simulink model "sharedControlWControllers"  (R2018a)
settings: Solver=FixedStepAuto  StartTime=0.0  StopTime=500  FixedStep=.1  RelTol=1e-3
values from neighbouring files (symbols this model uses):
  a = -real(s1) + imag(s1)/tan(angle(s1+b) - theta)    [RLDesignJoystick.m]    (also in gainPlot.m = 10)
  a1 = b1/K    [RLDesignJoystick.m]
  b = 1.2*bb/I    (= 0.4)    [RLDesignJoystick.m]    (also in gainPlot.m)
  b1 = -real(s1)/150    [RLDesignJoystick.m]
  K0 = abs(s1+a)/abs(Gs1)/abs(s1+b)    [RLDesignJoystick.m]    (also in gainPlot.m = 0.5)
  K1 = 1/abs(Gs1)    [RLDesignJoystick.m]
undefined symbols (not defined in the file or in its folder): a2, b2, K2
libraries: simulink x2, commfilt2 x2
settings Model: Creator=transmogrifierlight  LastModifiedBy=thedoctor

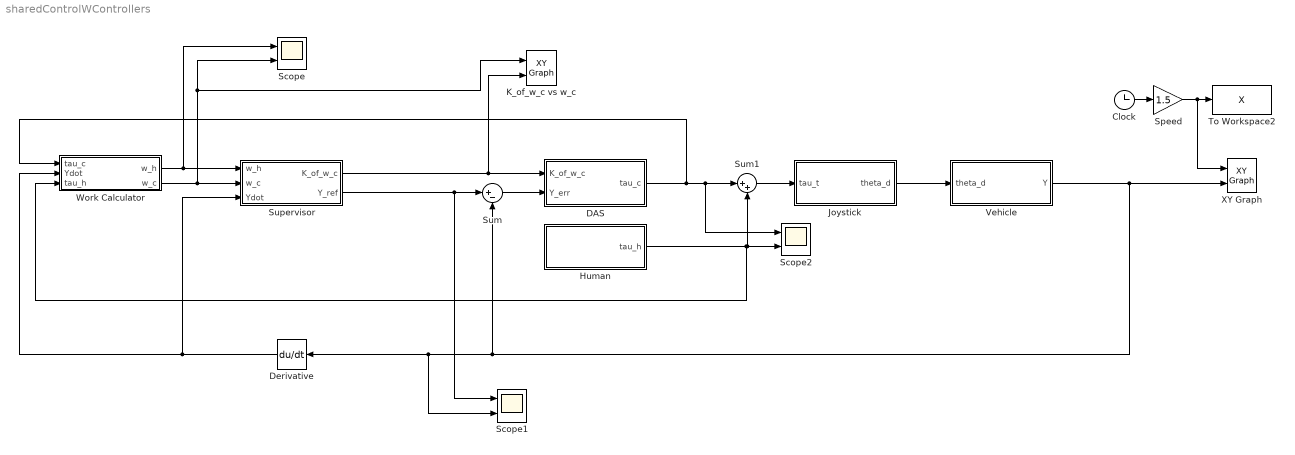
== system sharedControlWControllers ==
  Clock : Clock
  DAS : Subsystem
  Derivative : Derivative
  Human : Subsystem
  Joystick : Subsystem
  K_of_w_c vs w_c : simulink/Sinks/XY Graph  xmin=-01  xmax=2  ymin=-0.5  ymax=1  st=-1
  Scope : Scope  NumInputPorts=2
  Scope1 : Scope  NumInputPorts=2
  Scope2 : Scope  NumInputPorts=2
  Speed : Gain  Gain=1.5
  Sum : Sum  Inputs=|+-
  Sum1 : Sum  Inputs=|++
  Supervisor : Subsystem  mask{gamma_1_sq=0, gamma_2_sq=0, a_d=10, b_d=0.4, sigma_sq=0.3, delta_y=4, K0=0.5}
      mask prompts: gamma_1_sq "DAS Threshold"; gamma_2_sq "Human Threshold"; a_d "a"; b_d "b"; sigma_sq "Lane Change Threshold"; delta_y "Lane Change Delta"
  To Workspace2 : ToWorkspace  VariableName=X  SaveFormat=Timeseries  SampleTime=-1
  Vehicle : Subsystem
  Work Calculator : Subsystem
  XY Graph : simulink/Sinks/XY Graph  xmin=-10  xmax=1.5*1500  ymin=-100  ymax=100  st=-1
  wires:
  Work Calculator/1(w_h) -> Scope/1, Supervisor/1(w_h)
  Work Calculator/2(w_c) -> K_of_w_c vs w_c/1, Scope/2, Supervisor/2(w_c)
  Supervisor/1(K_of_w_c) -> K_of_w_c vs w_c/2, DAS/1("K_of_w_c ")
  Supervisor/2(Y_ref) -> Scope1/1, Sum/1
  Sum/1 -> DAS/2(Y_err)
  DAS/1(tau_c) -> Scope2/1, Sum1/1, Work Calculator/1(tau_c)
  Sum1/1 -> Joystick/1(tau_t)
  Clock/1 -> Speed/1
  Speed/1 -> XY Graph/1, To Workspace2/1
  Vehicle/1(Y) -> Sum/2, Scope1/2, Derivative/1, XY Graph/2
  Derivative/1 -> Supervisor/3(Ydot), Work Calculator/2(Ydot)
  Joystick/1(theta_d) -> Vehicle/1(theta_d)
  Human/1(tau_h) -> Work Calculator/3(tau_h), Sum1/2, Scope2/2

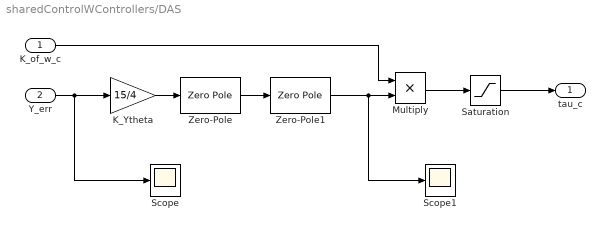
== system sharedControlWControllers/DAS ==
  "K_of_w_c " : Inport
  Y_err : Inport  Port=2
  K_Ytheta : Gain  Gain=15/4
  Multiply : Product
  Saturation : Saturate  UpperLimit=3.5  LowerLimit=-3.5
  Scope : Scope
  Scope1 : Scope
  Zero-Pole : ZeroPole  Zeros=[-b]  Poles=[-a]  Gain=[K0]
  Zero-Pole1 : ZeroPole  Zeros=[-b1]  Poles=[-a1]  Gain=[K1]
  tau_c : Outport
  wires:
  Y_err/1 -> Scope/1, K_Ytheta/1
  Saturation/1 -> tau_c/1
  Multiply/1 -> Saturation/1
  "K_of_w_c "/1 -> Multiply/1
  K_Ytheta/1 -> Zero-Pole/1
  Zero-Pole1/1 -> Scope1/1, Multiply/2
  Zero-Pole/1 -> Zero-Pole1/1

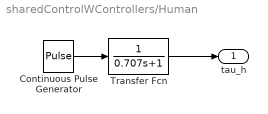
== system sharedControlWControllers/Human ==
  Continuous Pulse Generator : DiscretePulseGenerator  PulseType=Time based  Amplitude=3.5  Period=100  PhaseDelay=30
  Transfer Fcn : TransferFcn  Denominator=[0.707 1]
  tau_h : Outport
  wires:
  Transfer Fcn/1 -> tau_h/1
  Continuous Pulse Generator/1 -> Transfer Fcn/1

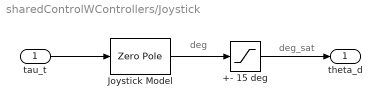
== system sharedControlWControllers/Joystick ==
  note: deg_sat
  note: deg
  tau_t : Inport
  +- 15 deg : Saturate  UpperLimit=15  LowerLimit=-15
  Joystick Model : ZeroPole  Zeros=[]  Poles=[0 -0.254/0.762]  Gain=[0.762]
  theta_d : Outport
  wires:
  Joystick Model/1 -> +- 15 deg/1
  +- 15 deg/1 -> theta_d/1
  tau_t/1 -> Joystick Model/1

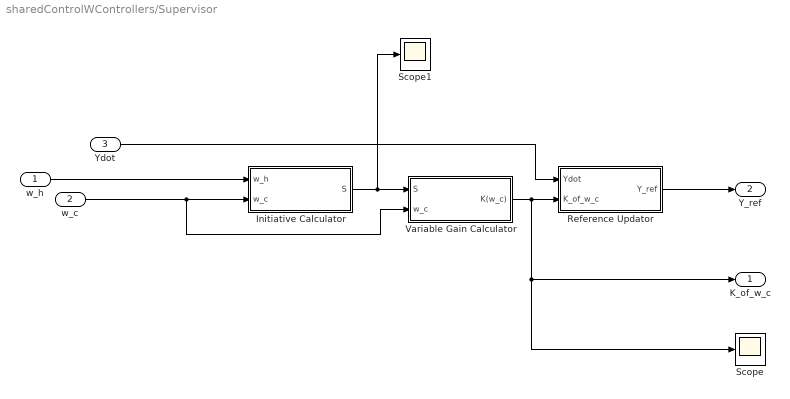
== system sharedControlWControllers/Supervisor ==
  w_h : Inport
  w_c : Inport  Port=2
  Ydot : Inport  Port=3
  Initiative Calculator : Subsystem
  Reference Updator : Subsystem
  Scope : Scope
  Scope1 : Scope
  Variable Gain Calculator : Subsystem
  K_of_w_c : Outport
  Y_ref : Outport  Port=2
  wires:
  w_c/1 -> Variable Gain Calculator/2(w_c), Initiative Calculator/2("w_c ")
  w_h/1 -> Initiative Calculator/1(w_h)
  Initiative Calculator/1(S) -> Scope1/1, Variable Gain Calculator/1(S)
  Variable Gain Calculator/1(K(w_c)) -> Reference Updator/2(K_of_w_c), Scope/1, K_of_w_c/1
  Ydot/1 -> Reference Updator/1(Ydot)
  Reference Updator/1(Y_ref) -> Y_ref/1

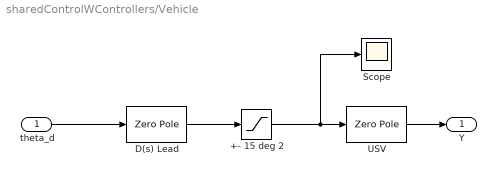
== system sharedControlWControllers/Vehicle ==
  theta_d : Inport
  +- 15 deg 2 : Saturate  UpperLimit=15  LowerLimit=-15
  D(s) Lead : ZeroPole  Zeros=[-b2]  Poles=[-a2]  Gain=[K2]
  Scope : Scope
  USV : ZeroPole  Zeros=[]  Poles=[0 0 -5/4]  Gain=[1.5*1e-2]
  Y : Outport
  wires:
  +- 15 deg 2/1 -> Scope/1, USV/1
  USV/1 -> Y/1
  theta_d/1 -> D(s) Lead/1
  D(s) Lead/1 -> +- 15 deg 2/1

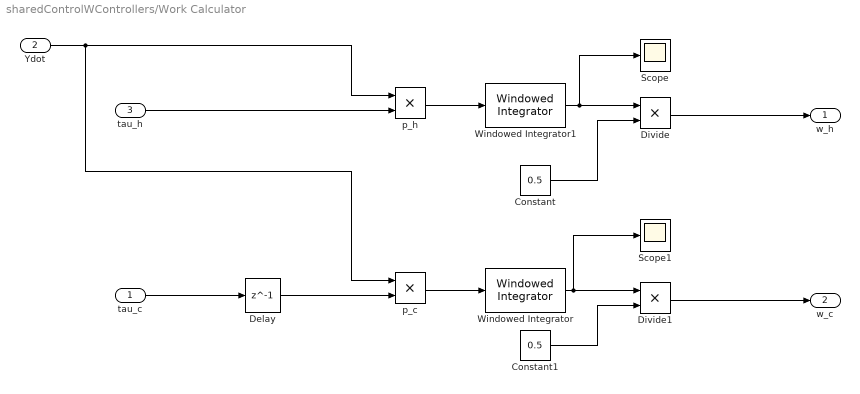
== system sharedControlWControllers/Work Calculator ==
  tau_c : Inport
  Ydot : Inport  Port=2
  tau_h : Inport  Port=3
  Constant : Constant  Value=0.5
  Constant1 : Constant  Value=0.5
  Delay : Delay  DelayLength=1
  Divide : Product
  Divide1 : Product
  Scope : Scope
  Scope1 : Scope
  Windowed Integrator : commfilt2/Windowed Integrator  integperiod=20  InputProcessing=Columns as channels (frame based)  roundingMode=Floor  overflowMode=off  coeffDataTypeStr=Inherit: Same word length as input  coeffMin=[]  coeffMax=[]  coeffLastDataTypeStr=Inherit: Same word length as input  accumDataTypeStr=Inherit: Same as product output  accumLastDataTypeStr=Inherit: Same as product output  outputDataTypeStr=Inherit: Same as accumulator  outputMin=[]  outputMax=[]  outputLastDataTypeStr=Inherit: Same as accumulator
      settings: SourceProductName=Communications System Toolbox  SourceProductBaseCode=CM
  Windowed Integrator1 : commfilt2/Windowed Integrator  integperiod=20  InputProcessing=Columns as channels (frame based)  roundingMode=Floor  overflowMode=off  coeffDataTypeStr=Inherit: Same word length as input  coeffMin=[]  coeffMax=[]  coeffLastDataTypeStr=Inherit: Same word length as input  accumDataTypeStr=Inherit: Same as product output  accumLastDataTypeStr=Inherit: Same as product output  outputDataTypeStr=Inherit: Same as accumulator  outputMin=[]  outputMax=[]  outputLastDataTypeStr=Inherit: Same as accumulator
      settings: SourceProductName=Communications System Toolbox  SourceProductBaseCode=CM
  p_c : Product
  p_h : Product
  w_h : Outport
  w_c : Outport  Port=2
  wires:
  Divide/1 -> w_h/1
  Ydot/1 -> p_c/1, p_h/1
  Constant/1 -> Divide/2
  p_h/1 -> Windowed Integrator1/1
  tau_h/1 -> p_h/2
  tau_c/1 -> Delay/1
  Windowed Integrator/1 -> Scope1/1, Divide1/1
  p_c/1 -> Windowed Integrator/1
  Constant1/1 -> Divide1/2
  Divide1/1 -> w_c/1
  Windowed Integrator1/1 -> Scope/1, Divide/1
  Delay/1 -> p_c/2

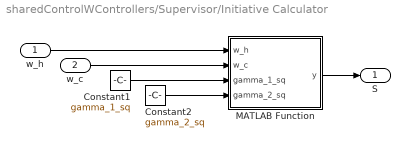
== system sharedControlWControllers/Supervisor/Initiative Calculator ==
  w_h : Inport
  "w_c " : Inport  Port=2
  Constant1 : Constant  Value=gamma_1_sq
  Constant2 : Constant  Value=gamma_2_sq
  MATLAB Function : MATLAB Function  TreatAsAtomicUnit=on
  S : Outport
  wires:
  w_h/1 -> MATLAB Function/1(w_h)
  MATLAB Function/1(y) -> S/1
  Constant2/1 -> MATLAB Function/4(gamma_2_sq)
  "w_c "/1 -> MATLAB Function/2(w_c)
  Constant1/1 -> MATLAB Function/3(gamma_1_sq)

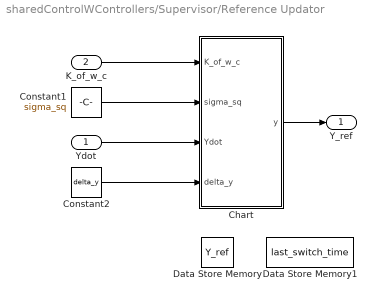
== system sharedControlWControllers/Supervisor/Reference Updator ==
  Ydot : Inport
  K_of_w_c : Inport  Port=2
  Chart : Stateflow chart  TreatAsAtomicUnit=on
  Constant1 : Constant  Value=sigma_sq
  Constant2 : Constant  Value=delta_y
  Data Store Memory : DataStoreMemory  DataStoreName=Y_ref  ReadBeforeWriteMsg=warning  WriteAfterWriteMsg=warning  WriteAfterReadMsg=warning  ShowAdditionalParam=off  OutDataTypeStr=int16
  Data Store Memory1 : DataStoreMemory  DataStoreName=last_switch_time  ReadBeforeWriteMsg=warning  WriteAfterWriteMsg=warning  WriteAfterReadMsg=warning  ShowAdditionalParam=off  OutDataTypeStr=double
  Y_ref : Outport
  wires:
  Ydot/1 -> Chart/3(Ydot)
  K_of_w_c/1 -> Chart/1(K_of_w_c)
  Chart/1(y) -> Y_ref/1
  Constant1/1 -> Chart/2(sigma_sq)
  Constant2/1 -> Chart/4(delta_y)

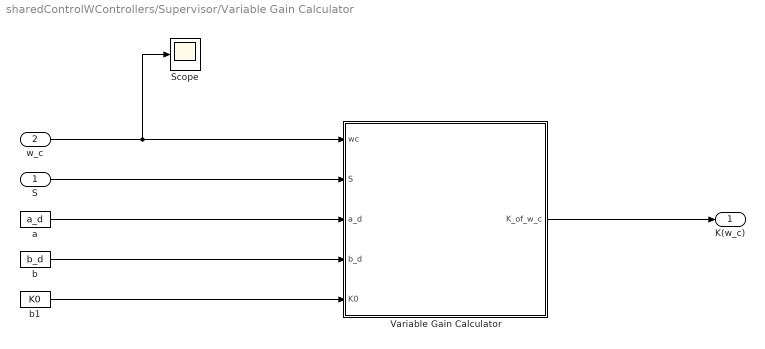
== system sharedControlWControllers/Supervisor/Variable Gain Calculator ==
  S : Inport
  w_c : Inport  Port=2
  Scope : Scope
  "Variable Gain Calculator " : MATLAB Function  TreatAsAtomicUnit=on
  a : Constant  Value=a_d
  b : Constant  Value=b_d
  b1 : Constant  Value=K0
  K(w_c) : Outport
  wires:
  "Variable Gain Calculator "/1(K_of_w_c) -> K(w_c)/1
  a/1 -> "Variable Gain Calculator "/3(a_d)
  w_c/1 -> Scope/1, "Variable Gain Calculator "/1(wc)
  S/1 -> "Variable Gain Calculator "/2(S)
  b/1 -> "Variable Gain Calculator "/4(b_d)
  b1/1 -> "Variable Gain Calculator "/5(K0)

== stateflow chart sharedControlWControllers/Supervisor/Reference Updator/Chart ==
  note: This system will check if there should be a lane changed
      | based on K(w_c) vs siqma^2.  If a lane change is required,
      | check to see if allowed based on time since last lane change
  note: C style logic:
      | if(K_of_w_c<=sigma_sq)
      | if(Ydot>0)
      | Y_ref=Y_ref+delta_y;
      | elseif(Ydot<0)
      | Y_ref=Y_ref-delta_y;
      | end
      | end
      | y = Y_ref;
  state add
    entry:Y_ref=Y_ref+delta_y;
    y=Y_ref;
    set_last_switch_time;
  state checkForChange
    entry: change_flag=time_check(10);
  state subtract
    entry:Y_ref=Y_ref-delta_y;
    y=Y_ref;
    set_last_switch_time;
  note: T_min=5
  add -> checkForChange
  (default) -> checkForChange
  (junction 47) -> add [order 1] : [Ydot>0]
  checkForChange -> (junction 44) [order 1] : [change_flag==true]
  (junction 44) -> (junction 47) [order 1] : [(K_of_w_c<=sigma_sq)]
  (junction 44) -> checkForChange [order 2] : [(K_of_w_c>sigma_sq)]
  (junction 47) -> subtract [order 2] : [Ydot<0]
  checkForChange -> checkForChange [order 2] : [change_flag==false]
  subtract -> checkForChange
  data: change function_output; t_min function_input; K_of_w_c input; sigma_sq input; y output; Ydot input; delta_y input; Y_ref data_store_memory; last_switch_time data_store_memory; current_time local; change_flag local
  function change=time_check(t_min):
    | function change=time_check(t_min)
    | global last_switch_time
    | coder.extrinsic('get_param');
    | temp=0;
    | temp=get_param('sharedControl3','SimulationTime')
    | change=(temp-last_switch_time)>t_min;
  function set_last_switch_time:
    | function set_last_switch_time
    | global last_switch_time
    | coder.extrinsic('get_param')
    | last_switch_time=get_param('sharedControl3','SimulationTime');

== matlab function sharedControlWControllers/Supervisor/Initiative Calculator/MATLAB Function ==
  data: w_h input; y output; w_c input; gamma_1_sq input; gamma_2_sq input
function y = fcn(w_h, w_c, gamma_1_sq, gamma_2_sq)

if(w_h >= -gamma_1_sq && w_c >= -gamma_2_sq)
    S=1;
elseif(w_h >= -gamma_1_sq && w_c < -gamma_2_sq)
    S=2;
elseif(w_h < -gamma_1_sq && w_c >= -gamma_2_sq)
    S=3;
elseif(w_h < -gamma_1_sq && w_c < -gamma_2_sq)
    S=4;
else
    error('bad state assignment');
end
y = S;

== matlab function sharedControlWControllers/Supervisor/Variable Gain Calculator/Variable Gain Calculator  ==
  data: wc input; S input; K_of_w_c output; a_d input; b_d input; K0 input
function K_of_w_c = fcn(wc, S, a_d, b_d, K0)

if S == 2    
    K_of_w_c = K0/(1 + exp(-a_d*wc + b_d));
else
    K_of_w_c = K0;
end

return
